simulink model "QESO_ASGSM"  (R2024b)
settings: Solver=ode4  StartTime=0.0  StopTime=10  FixedStep=0.004  RelTol=1e-3
undefined symbols (not defined in the file or in its folder): DiscIntNeverNeededParam, SampleTime
libraries: aerolibutil x8, simulink_extras x3, sharedutil x3, sharedtransform x3, matrix_library x2, simulink x1
settings Model: Creator=danyy  LastModifiedBy=danyy

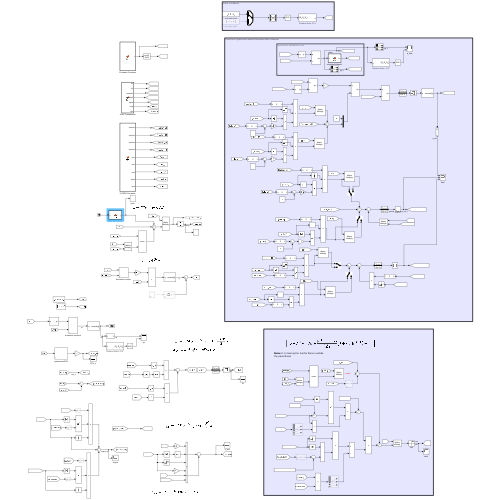
[thumbnail: Simulink's stored preview of the top-level diagram]
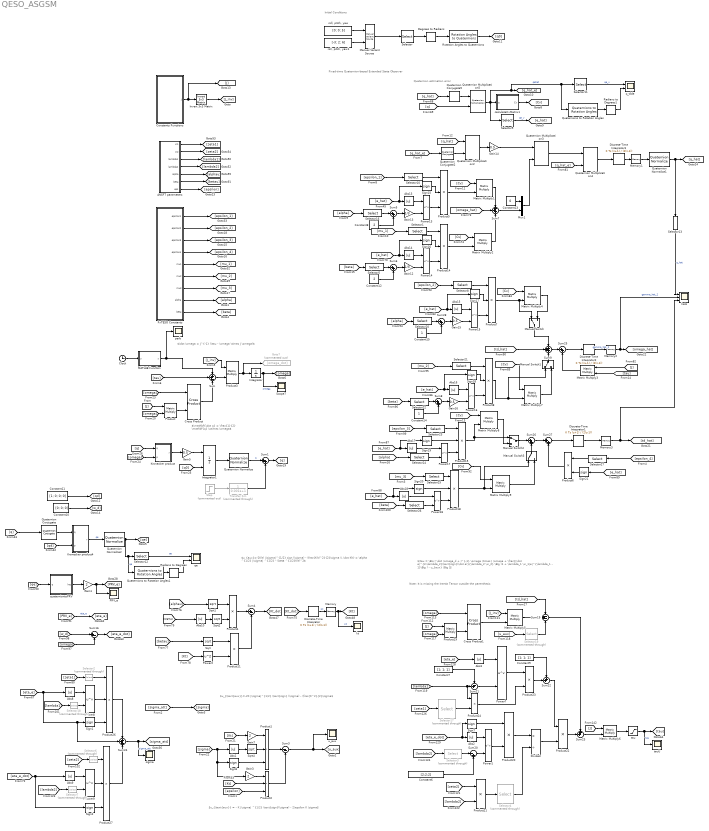
== system QESO_ASGSM ==
  note: $u_{\text{aux}} = - K |\sigma| ^{1/2} \text{sign}(\sigma) - 2\epsilon K \sigma$
  note: $u_{\text{aux}}=-2K |\sigma|^{1/2} \text{sign} (\sigma) - \frac{K^2}{2}\sigma$
  note: $u_{aux}=-2K(t) |\sigma|^{1/2} sign (\sigma) - \frac{K(t)^2}{2}\sigma \\ \dot K(t) = \alpha ^{1/2} |\sigma| ^{1/2} - \beta ^{1/2}K(t)^2$
  note: $\tau = \Big [ \dot \omega_d + J^{-1} \omega \times J \omega + \frac{|\dot e|^{2-\lambda_2}\text{sign}(\dot e)}{\lambda_2 \xi_2} \Big (1 + \lambda_1 \xi_1|e|^{\lambda_1 - 1}\Big ) - u_{aux} \Big ]$
  note: Note: It is missing the Inertia Tensor outside
      | the parenthesis
  note: $\mathbf{\dot q} = \frac{1}{2} \mathbf{q} \otimes \omega$
  note: $\dot \omega = J^{-1} (\tau - \omega \times J \omega)$
  note: Initial Conditions
  note: Fixed-time Quaternion-based Extended State Observer
  note: Quaternion estimation error
  ANSFT parameters : MATLAB Function  TreatAsAtomicUnit=on
  Abs{1..3,8..10,13..18} (12 alike) : Abs  SaturateOnIntegerOverflow=off
  Clock : Clock
  Constant10 : Constant  Value=[0; 0; 0]
  Constant11 : Constant  Value=[1; 0; 0; 0]
  Constant12 : Constant  Value=2
  Constant13 : Constant  Value=0
  Constant14 : Constant
  Constant15 : Constant
  Constant6 : Constant  Value=[2;2;2]
  Constant7 : Constant  Value=[1; 1; 1]
  Constant8 : Constant  Value=2
  Constant9 : Constant  Value=[1; 1; 1]
  Constants Functions : MATLAB Function  TreatAsAtomicUnit=on
  Cross Product : matrix_library/Cross Product
  Cross Product1 : matrix_library/Cross Product
  Degrees to Radians : simulink_extras/Transformations/Degrees to Radians
  Discrete-Time Integrator : DiscreteIntegrator  IntegratorMethod=Integration: Trapezoidal  InitialCondition=[0; 0; 0]  SampleTime=0.004  ICPrevOutput=DiscIntNeverNeededParam  ICPrevScaledInput=DiscIntNeverNeededParam
  Discrete-Time Integrator1 : DiscreteIntegrator  IntegratorMethod=Integration: Trapezoidal  InitialCondition=[0; 0; 0]  SampleTime=SampleTime  ICPrevOutput=DiscIntNeverNeededParam  ICPrevScaledInput=DiscIntNeverNeededParam
  Discrete-Time Integrator2 : DiscreteIntegrator  IntegratorMethod=Integration: Trapezoidal  InitialCondition=[0; 0; 0]  SampleTime=SampleTime  ICPrevOutput=DiscIntNeverNeededParam  ICPrevScaledInput=DiscIntNeverNeededParam
  Discrete-Time Integrator3 : DiscreteIntegrator  IntegratorMethod=Integration: Trapezoidal  InitialCondition=[1; 0; 0; 0]  SampleTime=SampleTime  ICPrevOutput=DiscIntNeverNeededParam  ICPrevScaledInput=DiscIntNeverNeededParam
  Divide3 : Product  Inputs=*/
  FxTESO Constants : MATLAB Function  TreatAsAtomicUnit=on
  Gain1 : Gain  Gain=2
  Gain12 : Gain  Gain=1/3
  Gain13 : Gain  Gain=1/3
  Gain{5,14..16} (4 alike) : Gain  Gain=0.5
  Gain3 : Gain  Gain=2
  Gain7 : Gain  Gain=2
  Goto7 : Goto  Commented=on  GotoTag=omega_dot
  Integrator : Integrator  InitialCondition=[0; 0; 0]
  Integrator1 : Integrator  InitialConditionSource=external
  Invert 3x3 Matrix : aerolibutil/Invert  3x3 Matrix
  Kronecker product : Subsystem
      mask Display: image('KroneckerProduct_1.svg');
  Kronecker product4 : Subsystem
  MATLAB Function : MATLAB Function  TreatAsAtomicUnit=on
  Manual Variant Source : simulink/Signal Routing/Manual Variant Source  NumChoices=2  LabelModeActiveChoice=V_1
  Manual Switch{,1..3} (4 alike) : ManualSwitch
  Matrix Multiply{1..9} (9 alike) : Product  Multiplication=Matrix(*)
  Memory : Memory  InitialCondition=[0; 0; 0]  InheritSampleTime=on
  Memory1 : Memory  InitialCondition=[1; 0; 0; 0]  InheritSampleTime=on
  Memory2 : Memory  InitialCondition=[0; 0; 0]  InheritSampleTime=on
  Memory3 : Memory  InitialCondition=[0; 0; 0]  InheritSampleTime=on
  Mux1 : Mux  Inputs=2
  PRV_e : Scope
  Power{1,7..9,13..18} (10 alike) : Math  Operator=pow
  Power2 : Math  Operator=square
  Product : Product  Multiplication=Matrix(*)
  Product{1..2,5,7..8,14..15,18,26..27} (10 alike) : Product  Inputs=3
  Product{4,6,11,20..24} (8 alike) : Product
  Product19 : Product  Multiplication=Matrix(*)
  Product3 : Product  Multiplication=Matrix(*)
  Quaternion Conjugate : aerolibutil/Quaternion Conjugate
  Quaternion Conjugate2 : aerolibutil/Quaternion Conjugate
  Quaternion Conjugate5 : aerolibutil/Quaternion Conjugate
  Quaternion Multiplication{2..5} (4 alike) : aerolibutil/Quaternion Multiplication
  Quaternion Normalize : sharedutil/Quaternion Normalize  aMode=aMode
  Quaternion Normalize1 : sharedutil/Quaternion Normalize  aMode=aMode
  Quaternion Normalize2 : sharedutil/Quaternion Normalize  aMode=aMode
  Quaternions to Rotation Angles : sharedtransform/Quaternions to Rotation Angles  rotationOrder=XYZ  aMode=aMode
  Quaternions to Rotation Angles1 : sharedtransform/Quaternions to Rotation Angles  rotationOrder=XYZ  aMode=aMode
  Radians to Degrees : simulink_extras/Transformations/Radians to Degrees
  Radians to Degrees1 : simulink_extras/Transformations/Radians to Degrees
  Rotation Angles to Quaternions : sharedtransform/Rotation Angles to Quaternions  rotationOrder=ZYX  aMode=aMode
  Scope7 : Scope
  Selector : Selector  InputPortWidth=3  IndexOptions=Index vector (dialog)  Indices=[3 2 1]  OutputSizes=1
  Selector{1,5,8,10,16,20..27} (13 alike) : Selector  InputPortWidth=6  IndexOptions=Index vector (dialog)  Indices=[4:6]  OutputSizes=1
  Selector{9,11..13} (4 alike) : Selector  InputPortWidth=4  IndexOptions=Index vector (dialog)  Indices=[2:4]  OutputSizes=1
  Selector{2..4,6..7,17..19} (8 alike) : Selector  Commented=through  InputPortWidth=6  IndexOptions=Index vector (dialog)  Indices=[4:6]  OutputSizes=1
  Sign{1..2,7..8,15..21} (11 alike) : Signum
  Sqrt{,1..2,4} (4 alike) : Sqrt
  Step : Step  Commented=on  Time=5  Before=[0; 0; 0; 0]  After=[0; 0; 0; 0.03]  SampleTime=0
  Sum : Sum  Inputs=++-
  Sum{1,5..6,8,25..28} (8 alike) : Sum  Inputs=|++
  Sum16 : Sum  Inputs=|+-
  Sum19 : Sum  Inputs=-+-
  Sum20 : Sum  Inputs=|-+
  Sum21 : Sum  Inputs=-+|
  Sum22 : Sum  Inputs=++|
  Sum23 : Sum  Inputs=++|
  Sum24 : Sum  Inputs=+++
  Sum3 : Sum  Inputs=|--
  Sum4 : Sum  Inputs=|+-
  Sum7 : Sum  Inputs=+++
  Sum9 : Sum  Inputs=+++
  Transfer Fcn : TransferFcn  Commented=through  Denominator=[0.001 1]
  calculateCvMatrix1 : MATLAB Function  TreatAsAtomicUnit=on
  hats : Scope  NumInputPorts=3
  kt : Scope
  perb : Scope
  q_tilde : Scope  NumInputPorts=2
  qe : Scope  NumInputPorts=2
  quaterniontoPRV : Subsystem
  "roll, pitch, yaw" : Constant  Value=[0; 0; 5]
  "roll, pitch, yaw1" : Constant  Value=[-3; 2; 6]
  sigma : Scope
  tau : Saturate
  tauU : Scope
  u_aux : Scope
  wires:
  Kronecker product4/1(r) -> Quaternion Normalize2/1  "qe"
  [qd] -> Kronecker product4/2(p)
  quaterniontoPRV/1(lnq) -> Gain1/1
  Quaternion Normalize2/1 -> Quaternions to Rotation Angles1/1, Selector12/1, [qe]  "qe"
  Quaternion Conjugate/1 -> Kronecker product4/1(q)
  [q] -> Quaternion Conjugate/1
  [qe] -> quaterniontoPRV/1(q)
  Gain1/1 -> PRV_e/1, [PRV_e]
  [PRV_e] -> [eta_e]  "eta_e"
  [w_d] -> Sum16/1
  [omega] -> Sum16/2
  Sum16/1 -> [eta_e_dot]
  Product27/1 -> Sum24/3
  Selector18/1 -> Power8/2
  Selector6/1 -> Product27/1
  [eta_e] -> Sum24/2, Sign1/1, Abs8/1
  Selector7/1 -> Power9/2
  Abs8/1 -> Power8/1
  [eta_e_dot] -> Abs9/1, Sign2/1
  [lambda2] -> Selector7/1
  [lambda1] -> Selector18/1
  Product26/1 -> Sum24/1
  [zeta2] -> Selector6/1
  Abs9/1 -> Power9/1
  [zeta1] -> Selector2/1
  Sum24/1 -> sigma/1, [sigma_att]  "sigma_att"
  Selector2/1 -> Product26/1
  Sign2/1 -> Product27/3
  Power9/1 -> Product27/2
  Sign1/1 -> Product26/3
  Power8/1 -> Product26/2
  Gain3/1 -> Product2/1
  Sum4/1 -> [Kt_dot]
  Sum3/1 -> u_aux/1, [u_aux]
  [Kt_dot] -> Discrete-Time Integrator/1
  [Kt] -> Power2/1
  [betau] -> Sqrt/1
  Product11/1 -> Sum4/2
  Product2/1 -> Sum3/2
  [Kt] -> Gain7/1
  [sigma_att] -> [sigma]
  Sign8/1 -> Product1/3
  Sqrt1/1 -> Product4/1
  [alphau] -> Sqrt1/1
  Power2/1 -> Product11/2
  Memory/1 -> kt/1, [Kt]  "Kt"
  Gain7/1 -> Product1/1
  [sigma] -> Abs10/1
  [epsilon] -> Product2/3
  Product1/1 -> Sum3/1
  Abs10/1 -> Sqrt2/1
  Product4/1 -> Sum4/1
  Sqrt/1 -> Product11/1
  Sqrt2/1 -> Product4/2
  Discrete-Time Integrator/1 -> Memory/1  "Kt"
  [Kt] -> Product2/2
  Sqrt4/1 -> Product1/2
  [sigma] -> Abs1/1, Gain3/1, Sign8/1
  Abs1/1 -> Sqrt4/1
  Product23/1 -> Sum22/2
  Sum22/1 -> Product22/1
  Product20/1 -> Divide3/1
  [td_hat] -> Sum19/1
  Matrix Multiply5/1 -> ?
  Matrix Multiply6/1 -> tau/1
  [lambda2] -> Selector3/1
  Product21/1 -> Selector4/1
  Sum21/1 -> Power7/2
  [lambda1] -> Product24/1, Sum21/2
  Constant9/1 -> Sum22/1
  [J_inv] -> Matrix Multiply5/1
  [J] -> Product19/1
  [u_aux] -> Selector19/1
  Product19/1 -> Cross Product1/2
  [lambda2] -> Product21/2
  tau/1 -> tauU/1, [tau]  "tau"
  Sum23/1 -> Matrix Multiply6/2
  Constant6/1 -> Sum20/2
  [eta_e_dot] -> Sign7/1, Abs2/1
  Cross Product1/1 -> Matrix Multiply5/2
  Selector19/1 -> Sum19/3
  Selector4/1 -> Divide3/2
  [eta_e] -> Abs3/1
  Sum19/1 -> Sum23/1
  [omega] -> Product19/2
  [zeta2] -> Product21/1
  Abs2/1 -> Power1/1
  Constant7/1 -> Sum21/1
  Power7/1 -> Product23/1
  Selector17/1 -> Product24/2
  [J] -> Matrix Multiply6/1
  [omega] -> Cross Product1/1
  Sum20/1 -> Power1/2
  Sign7/1 -> Product20/1
  Product22/1 -> Sum23/2
  [zeta1] -> Selector17/1
  Product24/1 -> Product23/2
  Selector3/1 -> Sum20/1
  Divide3/1 -> Product22/2
  Power1/1 -> Product20/2
  Abs3/1 -> Power7/1
  Product3/1 -> Goto7/1, Integrator/1
  [omega] -> Cross Product/1
  Sum/1 -> Product3/2
  [omega] -> Product/2
  Product/1 -> Cross Product/2
  Cross Product/1 -> Sum/3
  Integrator/1 -> Scope7/1, [omega]  "omega"
  [tau] -> Sum/2
  [J_inv] -> Product3/1
  [J] -> Product/1
  Selector/1 -> Degrees to Radians/1
  Rotation Angles to Quaternions/1 -> [q0]
  "roll, pitch, yaw1"/1 -> Manual Variant Source/2
  "roll, pitch, yaw"/1 -> Manual Variant Source/1
  Manual Variant Source/1 -> Selector/1
  Degrees to Radians/1 -> Rotation Angles to Quaternions/1
  Constants Functions/1(J) -> [J], Invert 3x3 Matrix/1
  Invert 3x3 Matrix/1 -> [J_inv]
  ANSFT parameters/2(xi2) -> [zeta2]
  ANSFT parameters/6(beta) -> [betau]
  ANSFT parameters/1(xi1) -> [zeta1]
  ANSFT parameters/5(alpha) -> [alphau]
  ANSFT parameters/4(lambda2) -> [lambda2]
  ANSFT parameters/3(lambda1) -> [lambda1]
  Constant10/1 -> [w_d]
  Constant11/1 -> [qd]
  ANSFT parameters/7(eps) -> [epsilon]
  Constant15/1 -> Sum28/2
  Selector1/1 -> Product14/1
  Matrix Multiply4/1 -> Manual Switch/2
  Sign20/1 -> Product18/2
  Memory2/1 -> hats/2, [omega_hat]  "gamma_hat_2"
  [e_hat] -> Sign15/1, Abs13/1
  [epsilon_1] -> Selector10/1
  Quaternion Multiplication2/1 -> Gain14/1
  [Cv] -> Matrix Multiply9/1
  Selector8/1 -> Product7/1
  [e_hat] -> Sign21/1
  Discrete-Time Integrator2/1 -> Memory2/1  "gamma_hat_2"
  [alpha] -> Selector16/1
  Sum9/1 -> Sum25/1
  Abs15/1 -> Power15/1
  [epsilon_4] -> Selector27/1
  [beta] -> Selector22/1
  Power16/1 -> Product8/3
  Power18/1 -> Product18/3
  [Cv] -> Matrix Multiply4/1
  Sign15/1 -> Product5/2
  Power13/1 -> Product5/3
  Mux1/1 -> Quaternion Multiplication3/2
  [tau] -> Matrix Multiply3/2
  Constant12/1 -> Sum6/2
  Gain16/1 -> Power16/2
  [e_hat] -> Sign16/1, Abs14/1
  Quaternion Multiplication3/1 -> Quaternion Multiplication4/1
  Product6/1 -> Sum27/2
  Quaternion Conjugate5/1 -> Quaternion Multiplication5/1
  Memory1/1 -> Quaternion Normalize1/1
  [e_hat] -> Sign18/1, Abs16/1
  [beta] -> Selector26/1
  Selector23/1 -> Product15/1
  Constant8/1 -> Sum5/2
  Quaternion Conjugate2/1 -> Quaternion Multiplication2/2
  Power17/1 -> Product15/3
  Gain15/1 -> Power15/2
  [q_hat] -> Quaternion Conjugate5/1
  Constant13/1 -> Mux1/1
  [mu_1] -> Selector1/1
  Matrix Multiply7/1 -> Manual Switch1/2
  Gain12/1 -> Power14/2
  Sign17/1 -> Product7/2
  Product8/1 -> Matrix Multiply7/2, Manual Switch1/1
  Quaternion Normalize1/1 -> Selector13/1, [q_hat]
  [q_hat_e] -> Quaternion Conjugate2/1
  [epsilon_2] -> Selector8/1
  [alpha] -> Selector24/1
  [alpha] -> Selector20/1
  Sum6/1 -> Gain12/1
  [e_hat] -> Abs18/1, Sign20/1
  [omega_hat] -> Sum7/2
  Product5/1 -> Matrix Multiply1/2
  Sum7/1 -> Mux1/2
  Selector5/1 -> Sum6/1
  Power15/1 -> Product7/3
  Matrix Multiply8/1 -> Manual Switch2/2
  [epsilon_3] -> Selector23/1
  [e_hat] -> Sign17/1, Abs15/1
  Abs14/1 -> Power14/1
  [beta] -> Selector5/1
  Gain14/1 -> Quaternion Multiplication3/1
  [q_hat_e] -> Quaternion Multiplication4/2
  Selector16/1 -> Sum5/1
  Product7/1 -> Manual Switch/1, Matrix Multiply4/2
  Selector21/1 -> Product8/1
  Sum5/1 -> Gain13/1
  [q_hat] -> Quaternion Multiplication2/1
  Selector27/1 -> Product6/1
  Sum26/1 -> Sum27/1
  [q] -> Quaternion Multiplication5/2
  Matrix Multiply2/1 -> Sum7/3
  [Cv] -> Matrix Multiply1/1
  [td_hat] -> Sum9/2
  Sign19/1 -> Product15/2
  Product15/1 -> Manual Switch2/1, Matrix Multiply8/2
  Product14/1 -> Matrix Multiply2/2
  [mu_2] -> Selector21/1
  Sign16/1 -> Product14/2
  Abs13/1 -> Power13/1
  [Cv] -> Matrix Multiply2/1
  Sum28/1 -> Gain15/1
  Selector20/1 -> Sum28/1
  calculateCvMatrix1/1(Cv) -> [Cv]
  Quaternion Multiplication5/1 -> Selector9/1, calculateCvMatrix1/1(q), Quaternions to Rotation Angles/1, Selector11/1, [q_hat_e]  "qehat"
  Selector22/1 -> Sum8/1
  Selector9/1 -> [e_hat]  "qe_v"
  Abs18/1 -> Power18/1
  Selector25/1 -> Product18/1
  Power14/1 -> Product14/3
  Memory3/1 -> hats/3, [td_hat]
  Abs16/1 -> Power16/1
  Sum25/1 -> Discrete-Time Integrator2/1
  Product18/1 -> Matrix Multiply9/2, Manual Switch3/1
  Sign18/1 -> Product8/2
  Matrix Multiply1/1 -> Sum7/1
  [Cv] -> Matrix Multiply8/1
  Quaternion Multiplication4/1 -> Discrete-Time Integrator3/1
  Discrete-Time Integrator1/1 -> Memory3/1
  Selector24/1 -> Power17/2
  Sign21/1 -> Product6/2
  Gain13/1 -> Power13/2
  Sum8/1 -> Gain16/1
  Discrete-Time Integrator3/1 -> Memory1/1
  Selector10/1 -> Product5/1
  Constant14/1 -> Sum8/2
  Matrix Multiply9/1 -> Manual Switch3/2
  Abs17/1 -> Power17/1
  Selector26/1 -> Power18/2
  [e_hat] -> Abs17/1, Sign19/1
  Matrix Multiply3/1 -> Sum25/2
  [mu_3] -> Selector25/1
  [J] -> Matrix Multiply3/1
  Sum27/1 -> Discrete-Time Integrator1/1
  [Cv] -> Matrix Multiply7/1
  FxTESO Constants/1(epsilon1) -> [epsilon_1]
  FxTESO Constants/9(beta) -> [beta]
  FxTESO Constants/2(epsilon2) -> [epsilon_2]
  FxTESO Constants/3(epsilon3) -> [epsilon_3]
  FxTESO Constants/8(alpha) -> [alpha]
  FxTESO Constants/5(mu1) -> [mu_1]
  FxTESO Constants/4(epsilon4) -> [epsilon_4]
  FxTESO Constants/6(mu2) -> [mu_2]
  FxTESO Constants/7(mu3) -> [mu_3]
  Quaternion Normalize/1 -> Sum1/1  "q"
  [omega] -> Kronecker product/2(p)
  [q] -> Kronecker product/1(q)
  [q0] -> Integrator1/2
  Integrator1/1 -> Quaternion Normalize/1
  Gain5/1 -> Integrator1/1
  Kronecker product/1(r) -> Gain5/1
  Manual Switch/1 -> Sum9/1
  Manual Switch1/1 -> Sum9/3
  Manual Switch2/1 -> Sum26/1
  Manual Switch3/1 -> Sum26/2
  Selector11/1 -> q_tilde/1  "qe_v"
  Selector12/1 -> qe/1  "qe"
  Selector13/1 -> hats/1  "q_hat"
  Quaternions to Rotation Angles/1 -> Radians to Degrees1/1
  Quaternions to Rotation Angles1/1 -> Radians to Degrees/1
  Radians to Degrees/1 -> qe/2
  Radians to Degrees1/1 -> q_tilde/2
  Sum1/1 -> [q]
  Step/1 -> Transfer Fcn/1
  Transfer Fcn/1 -> Sum1/2
  MATLAB Function/1(y) -> perb/1, Sum/1
  Clock/1 -> MATLAB Function/1(u)

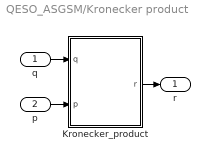
== system QESO_ASGSM/Kronecker product ==
  q : Inport
  p : Inport  Port=2
  Kronecker_product : MATLAB Function  TreatAsAtomicUnit=on
  r : Outport
  wires:
  q/1 -> Kronecker_product/1(q)
  p/1 -> Kronecker_product/2(p)
  Kronecker_product/1(r) -> r/1

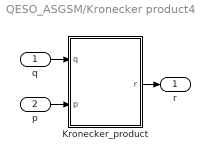
== system QESO_ASGSM/Kronecker product4 ==
  q : Inport
  p : Inport  Port=2
  Kronecker_product : MATLAB Function  TreatAsAtomicUnit=on
  r : Outport
  wires:
  q/1 -> Kronecker_product/1(q)
  p/1 -> Kronecker_product/2(p)
  Kronecker_product/1(r) -> r/1

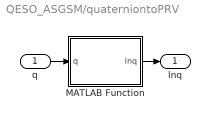
== system QESO_ASGSM/quaterniontoPRV ==
  q : Inport
  MATLAB Function : MATLAB Function  TreatAsAtomicUnit=on
  lnq : Outport
  wires:
  MATLAB Function/1(lnq) -> lnq/1
  q/1 -> MATLAB Function/1(q)

== matlab function QESO_ASGSM/MATLAB Function ==
  data: u input; y output
function y = fcn(u)

if (u < pi)
    y = [0; 0; 0];
else
    y = [0; 0; 0.02 * sin(u * 1 + pi)];
end

== matlab function QESO_ASGSM/Kronecker product/Kronecker_product ==
  data: q input; r output size=[4 1]; p input
function r = fcn(q, p)

%{
    Function to describe in matrix math the Kronecker product between
    two quaternions
    
    r = p kronecker q
    %}

    len = length(p);

    if len == 3 && length(q) == 4
        p1 = [0; p];
        q0 = q(1);
        q1 = q(2);
        q2 = q(3);
        q3 = q(4);
        
        % skew symmetric matrix
        q_matrix = [q0, -q1, -q2, -q3;
                  q1, q0, -q3, q2;
                  q2, q3, q0, -q1;
                  q3, -q2, q1, q0];
        
        r = q_matrix * p1;

    elseif len == 4
        q0 = q(1);
        q1 = q(2);
        q2 = q(3);
        q3 = q(4);
        
        % skew symmetric matrix
        q_matrix = [q0, -q1, -q2, -q3;
                  q1, q0, -q3, q2;
                  q2, q3, q0, -q1;
                  q3, -q2, q1, q0];
        
        r = q_matrix * p;

    else
        error('Quaternions dimensions do not match')
    end

== matlab function QESO_ASGSM/Constants Functions ==
  data: J output
function J  = fcn



% Jxx =  0.0411; % kg m²
% Jyy = 0.0478; % kg m²
% Jzz = 0.0599; % kg m²

Jxx = 0.028;
Jyy = 0.031;
Jzz = 0.048;

J = [Jxx, 0, 0;
     0, Jyy, 0;
     0, 0, Jzz];

== matlab function QESO_ASGSM/FxTESO Constants ==
  data: epsilon1 output; epsilon2 output; epsilon3 output; epsilon4 output; mu1 output; mu2 output; mu3 output; alpha output; beta output
function [epsilon1, epsilon2, epsilon3, epsilon4, mu1, mu2, mu3, alpha, beta] = fcn

% epsilon1 = [16; 16; 16; 16; 16; 12];
% epsilon2 = [150; 150; 175; 175; 175; 100];
% epsilon3 = [450; 450; 300; 300; 300; 250];
% 
% epsilon4 = [0.01, 0.01, 0.01, 0.001, 0.001, 0.05]';
% 
% mu1 = epsilon1;
% mu2 = epsilon2;
% mu3 = epsilon3;
% 
% alpha = [0.6; 0.6; 0.6; 0.7; 0.7; 0.7];
% 
% beta = [1.2; 1.2; 1.2; 1.2; 1.2; 1.2];

%% FxTESO-ASGSM

% epsilon1 = [16; 16; 16; 16; 16; 16];
% epsilon2 = [150; 150; 175; 175; 150; 150];
% epsilon3 = [450; 450; 500; 450; 450; 450];
% 
epsilon1 = [16; 16; 24; 16; 16; 20];
epsilon2 = [300; 300; 300; 300; 300; 375];
epsilon3 = [600; 600; 500; 600; 600; 575];

epsilon4 = [0.01, 0.01, 0.01, 0.01, 0.01, 0.005]';

mu1 = epsilon1;
mu2 = epsilon2;
mu3 = epsilon3;

alpha = [0.6; 0.6; 0.4; 0.6; 0.6; 0.65];

beta = [1.2; 1.2; 1.2; 1.2; 1.2; 1.2];

== matlab function QESO_ASGSM/quaterniontoPRV/MATLAB Function ==
  data: q input; lnq output size=[3 1]
function lnq = fcn(q)

if length(q) == 4
    q0 = q(1);
    q_vec = [q(2); q(3); q(4)];

    if norm(q_vec) == 0
        lnq = [0; 0; 0];
    else
        % q0 = real(q0);
        lnq = (q_vec / (norm(q_vec)) ) * acos(q0);
    end
else
    error('Input must be a vector 4 by 1 (Quaternion)')
end

== matlab function QESO_ASGSM/Kronecker product4/Kronecker_product ==
  data: q input; r output size=[4 1]; p input
function r = fcn(q, p)

%{
    Function to describe in matrix math the Kronecker product between
    two quaternions
    
    r = p kronecker q
    %}

    len = length(p);

    if len == 3 && length(q) == 4
        p1 = [0; p];
        q0 = q(1);
        q1 = q(2);
        q2 = q(3);
        q3 = q(4);
        
        % skew symmetric matrix
        q_matrix = [q0, -q1, -q2, -q3;
                  q1, q0, -q3, q2;
                  q2, q3, q0, -q1;
                  q3, -q2, q1, q0];
        
        r = q_matrix * p1;

    elseif len == 4
        q0 = q(1);
        q1 = q(2);
        q2 = q(3);
        q3 = q(4);
        
        % skew symmetric matrix
        q_matrix = [q0, -q1, -q2, -q3;
                  q1, q0, -q3, q2;
                  q2, q3, q0, -q1;
                  q3, -q2, q1, q0];
        
        r = q_matrix * p;

    else
        error('Quaternions dimensions do not match')
    end

== matlab function QESO_ASGSM/ANSFT parameters ==
  data: xi1 output; xi2 output; lambda1 output; lambda2 output; alpha output; beta output; eps output
function [xi1, xi2, lambda1, lambda2, alpha, beta, eps] = fcn

%% Constantes de la Superficie deslizante
% zeta1 parecido a una ganancia proporcional
xi1 = [0.5; 0.5; 0.1];
%zeta2 parecido a una ganancia derivatida
xi2 = [1; 1; 0.5];
% lambda 1 > lambda2
lambda1 = [2; 2; 2];
% 1 < lambda2 < 2
lambda2 = [1.33; 1.33; 1.2];
%% Constantes del control auxiliar
%minimize sigma
alpha = [1; 1; 100];
%aumetnar control, aumentar energía del sistema
beta = [0.005; 0.005; 0.001];

eps = [0.1; 0.1; 0.1];

== matlab function QESO_ASGSM/calculateCvMatrix1 ==
  data: q input; Cv output
function Cv = fcn(q)

q0 = q(1);
q1 = q(2);
q2 = q(3);
q3 = q(4);

Cv = [q0, -q3, q2;
      q3, q0, -q1;
      -q2, q1, q0] * 0.5;

Cv = pinv(Cv);
